simulink model "Vehicle_definitivo_validazione_2"  (R2025b)
settings: Solver=ode4  StartTime=0.0  StopTime=30  FixedStep=0.001  RelTol=1e-3
undefined symbols (not defined in the file): car, new_lotus_bump, new_lotus_roll, new_lotus_steer, posRef, rad, s, Tau_1, Tau_2, Tau_3, Tau_4, yawRef
libraries: aerolibconvert2 x28, simulink_extras x16, simulink x12, slpidlib x2, mpclib x1
(part 1 of 13)
settings Model: PacingRate=10  Creator=loren  LastModifiedBy=miche
settings SolverCC: ZeroCrossControl=DisableAll

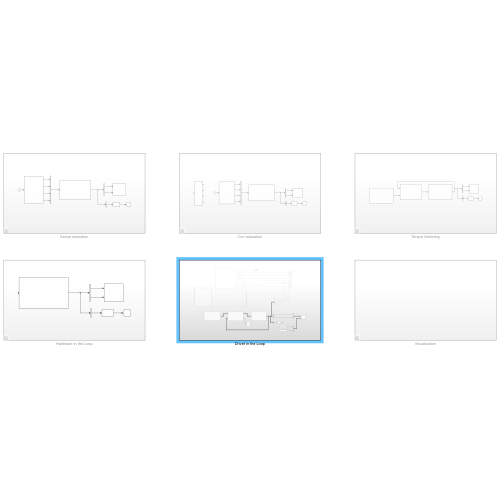
[thumbnail: Simulink's stored preview of the top-level diagram]
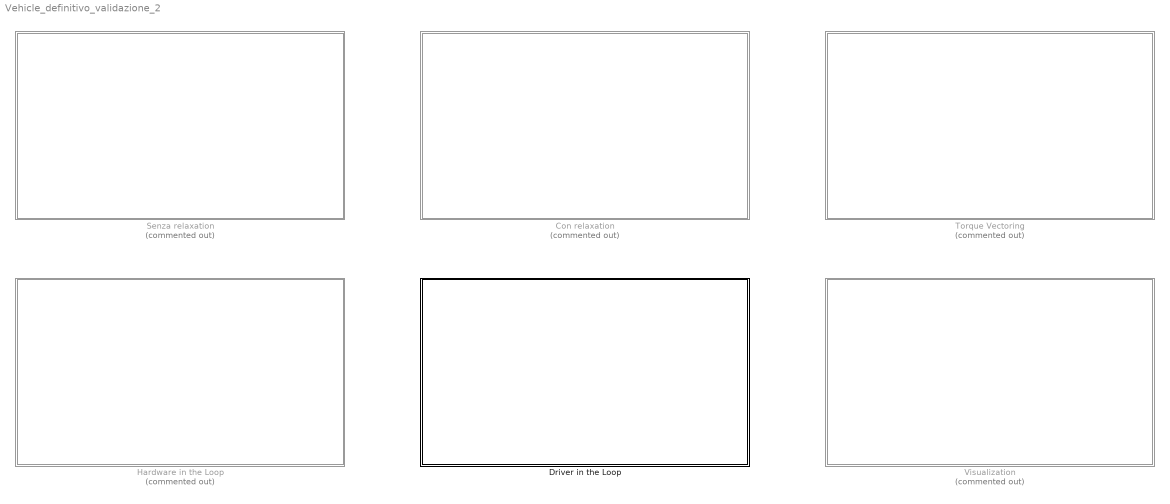
== system Vehicle_definitivo_validazione_2 ==
  Con relaxation : Subsystem  Commented=on
  Driver in the Loop : Subsystem
  Hardware in the Loop : Subsystem  Commented=on
  Senza relaxation : Subsystem  Commented=on
  Torque Vectoring : Subsystem  Commented=on
  Visualization : Subsystem  Commented=on

== system Vehicle_definitivo_validazione_2/Con relaxation ==
  Bus Creator : BusCreator  Inputs=4
  Bus Selector : BusSelector  OutputSignals=Veh_States.inertia_frame.X,Veh_States.inertia_frame.Y
  Bus Selector1 : BusSelector  OutputSignals=Veh_States.velocities.u
  Clock : Clock
  Compare To Constant3 : simulink/Logic and Bit Operations/Compare To Constant  relop=<=  const=2  OutDataTypeStr=boolean  ZeroCross=off
  MATLAB Function1 : MATLAB Function  TreatAsAtomicUnit=on
  MATLAB Function2 : MATLAB Function  TreatAsAtomicUnit=on
  Stop Simulation : Stop
  Vehicle : Subsystem
  XY Graph1 : Record  NumPorts=2.0  FileSettingsInternal="{\"entries\":[{\"content\":{\"excelSettings\":{\"content\":{},\"type\":\"Streamout.ExcelSettings\"},\"parquetSettings\":{\"content\":{},\"type\":\"Streamout.ParquetSettings\"}},\"type\":\"Streamout.FileSettingStorage\",\"uuid\":\"\"}],\"packageUris\":[\"http:\\/\\/schema.mathworks.com\\/mf0\\/streamout_blocks\\/R2020a\"],\"version\":\"1.0\"}"  FrameSettings=[0, 0]  Layout=[1 1]  SignalsInternal="{\"entries\":[{\"content\":{\"signals\":[{\"content\":{\"blockPath\":[],\"dimensions\":[1],\"domain\":\"\",\"lineColor\":\"#ff6929\",\"lineWidth\":2,\"port\":1,\"signalID\":1,\"signalName\":\"<X>\"},\"type\":\"RecordBlkView.Signal\",\"uuid\":\"\"},{\"content\":{\"blockPath\":[],\"dimensions\":[1],\"domain\":\"\",\"lineColor\":\"#b746ff\",\"lineWidth\":2,\"port\":2,\"signalID\":2,\"signalName\":\"<Y>\"},\"type\":\"RecordBlkView.Signal\",\"uuid\":\"\"}]},\"type\":\"RecordBlkView.InputSignals\",\"uuid\":\"\"}],\"packageUris\":[\"http:\\/\\/schema.mathworks.com\\/mf0\\/streamout_blocks\\/R2020a\"],\"version\":\"1.0\"}"  VisualizationBindings="{\"xyplotplugin\":{\"info\":[{\"series\":[],\"subplotID\":1}]}}"  CompatibilityTag=XY
  wires:
  Bus Creator/1 -> Vehicle/1(Driver)
  MATLAB Function2/4(bps) -> Bus Creator/4
  Clock/1 -> MATLAB Function2/1(t)
  MATLAB Function2/2(tps_ICE) -> Bus Creator/2
  Bus Selector1/1 -> Compare To Constant3/1  "<u>"
  MATLAB Function2/1(steer) -> Bus Creator/1
  Compare To Constant3/1 -> Stop Simulation/1
  Vehicle/1(Vehicle) -> Bus Selector1/1, Bus Selector/1  "Vehicle"
  MATLAB Function2/3(tps_EM) -> Bus Creator/3
  Bus Selector/1 -> XY Graph1/1  "<X>"
  Bus Selector/2 -> XY Graph1/2  "<Y>"

== system Vehicle_definitivo_validazione_2/Driver in the Loop ==
  Bus Creator : BusCreator  Inputs=2
  Bus Creator1 : BusCreator  Inputs=2
  Bus Creator2 : BusCreator  Commented=on  Inputs=4
  Bus Selector : BusSelector  OutputSignals=Veh_States.inertia_frame.X,Veh_States.inertia_frame.Y
  Bus Selector1 : BusSelector  OutputSignals=Veh_States.velocities.u
  Bus Selector2 : BusSelector  Commented=on  OutputSignals=Veh_States.velocities.u,Veh_States.accelerations.ax_prev,Veh_States.accelerations.ay_prev,Veh_States.velocities.v_tot
  Compare To Constant3 : simulink/Logic and Bit Operations/Compare To Constant  relop=<=  const=2  OutDataTypeStr=boolean  ZeroCross=off
  Constant : Constant  Commented=on  Value=0
  Constant1 : Constant  Commented=on  Value=0
  Driver : Subsystem
  From Workspace : FromWorkspace  VariableName=[t,posRef(:,1)]
  From Workspace1 : FromWorkspace  VariableName=[t,posRef(:,2)]
  From Spreadsheet : FromSpreadsheet  Commented=on  FileName=C:\Users\miche\Downloads\steer_fissato.xlsx  SheetName=Foglio1  Range=A3:H3989
  Gain : Gain  Commented=on  Gain=1/100
  Gain1 : Gain  Commented=on  Gain=-1
  Gain3 : Gain  Commented=on  Gain=1/3.6
  Gain4 : Gain  Commented=on  Gain=1/-9.81
  Gain7 : Gain  Commented=on  Gain=1/-9.81
  Lap Times : Display
  MATLAB Function versione 3 con memoria persistent1 : MATLAB Function  Commented=on  TreatAsAtomicUnit=on
  Scope : Scope
      settings: ActiveDisplayYMinimum=-1  ActiveDisplayYMaximum=1
  Scope1 : Scope  Commented=on
      settings: ActiveDisplayYMinimum=-1  ActiveDisplayYMaximum=1  DataLoggingVariableName=ScopeData6
  Scope2 : Scope  Commented=on
      settings: ActiveDisplayYMinimum=-89.125000000000455  ActiveDisplayYMaximum=-85.874999999999957  DataLoggingVariableName=ScopeData7
  Scope4 : Scope  Commented=on  NumInputPorts=3
      settings: ActiveDisplayYMinimum=2.9977159466940941  ActiveDisplayYMaximum=13.111056252836459  DataLoggingVariableName=ScopeData9
  Scope5 : Scope  Commented=on  NumInputPorts=2
      settings: ActiveDisplayYMinimum=-1.999530891220914  ActiveDisplayYMaximum=0.22217009902454593  DataLoggingVariableName=ScopeData10
  Scope6 : Scope  Commented=on  NumInputPorts=2
      settings: ActiveDisplayYMinimum=-1.1010446035915249  ActiveDisplayYMaximum=0.7997968068549437  DataLoggingVariableName=ScopeData11
  Stop Simulation : Stop
  Subsystem : Subsystem
  Terminator : Terminator
  Vehicle : Subsystem
  XY Graph : Record  NumPorts=2.0  FileSettingsInternal="{\"entries\":[{\"content\":{\"excelSettings\":{\"content\":{},\"type\":\"Streamout.ExcelSettings\"},\"parquetSettings\":{\"content\":{},\"type\":\"Streamout.ParquetSettings\"}},\"type\":\"Streamout.FileSettingStorage\",\"uuid\":\"\"}],\"packageUris\":[\"http:\\/\\/schema.mathworks.com\\/mf0\\/streamout_blocks\\/R2020a\"],\"version\":\"1.0\"}"  FrameSettings=[0, 0]  Layout=[1 1]  SignalsInternal="{\"entries\":[{\"content\":{\"signals\":[{\"content\":{\"blockPath\":[],\"dimensions\":[1],\"domain\":\"\",\"hasChildren\":true,\"lineColor\":\"#fe330a\",\"lineWidth\":2,\"port\":1,\"sid\":[\"\"],\"signalID\":1,\"signalName\":\"Bus\\nCreator\"},\"type\":\"RecordBlkView.Signal\",\"uuid\":\"\"},{\"content\":{\"blockPath\":[],\"dimensions\":[1],\"domain\":\"\",\"leafPath\":\"Bus\\nCreator.X\",\"lineColor\":\"#139fff\",\"lineWidth\":2,\"parentID\":1,\"plots\":[ 1 ],\"port\":1,\"sid\":[\"\"],\"signalID\":2,\"signalName\":\"Bus\\nCreator.X\"},\"type\":\"RecordBlkView.Signal\",\"uuid\":\"\"},{\"content\":{\"blockPath\":[],\"dimensions\":[1],\"domain\":\"\",\"leafPath\":\"Bus\\nCreator.Y\",\"lineColor\":\"#ff6929\",\"lineWidth\":2,\"parentID\":1,\"plots\":[ 1 ],\"port\":1,\"sid\":[\"\"],\"signalID\":3,\"signalName\":\"Bus\\nCreator.Y\"},\"type\":\"RecordBlkView.Signal\",\"uuid\":\"\"},{\"content\":{\"blockPath\":[],\"dimensions\":[1],\"domain\":\"\",\"hasChildren\":true,\"lineColor\":\"#d95319\",\"lineWidth\":2,\"port\":2,\"sid\":[\"\"],\"signalID\":4,\"signalName\":\"Bus\\nCreator1\"},\"type\":\"RecordBlkView.Signal\",\"uuid\":\"\"},{\"content\":{\"blockPath\":[],\"dimensions\":[1],\"domain\":\"\",\"leafPath\":\"Bus\\nCreator1.x_ref\",\"lineColor\":\"#fe330a\",\"lineWidth\":2,\"parentID\":4,\"plots\":[ 1 ],\"port\":2,\"sid\":[\"\"],\"signalID\":5,\"signalName\":\"Bus\\nCreator1.x_ref\"},\"type\":\"RecordBlkView.Signal\",\"uuid\":\"\"},{\"content\":{\"blockPath\":[],\"dimensions\":[1],\"domain\":\"\",\"leafPath\":\"Bus\\nCreator1.y_ref\",\"lineColor\":\"#22b573\",\"lineWidth\":2,\"parentID\":4,\"plots\":[ 1 ],\"port\":2,\"sid\":[\"\"],\"signalID\":6,\"signalName\":\"Bus\\nCreator1.y_ref\"},\"type\":\"RecordBlkView.Signal\",\"uuid\":\"\"}]},\"type\":\"RecordBlkView.InputSignals\",\"uuid\":\"\"}],\"packageUris\":[\"http:\\/\\/schema.mathworks.com\\/mf0\\/streamout_blocks\\/R2020a\"],\"version\":\"1.0\"}"  VisualizationBindings="{\"xyplotplugin\":{\"info\":[{\"series\":[{\"bindingParametersList\":[{\"parameter\":\"X-Axis\",\"signalID\":2,\"signalName\":\"Bus\\nCreator.X\"},{\"parameter\":\"Y-Axis\",\"signalID\":3,\"signalName\":\"Bus\\nCreator.Y\"}],\"seriesID\":0},{\"bindingParametersList\":[{\"parameter\":\"X-Axis\",\"signalID\":5,\"signalName\":\"Bus\\nCreator1.x_ref\"},{\"parameter\":\"Y-Axis\",\"signalID\":6,\"signalName\":\"Bus\\nCreator1.y_ref\"}],\"seriesID\":1}],\"subplotID\":1}]}}"  CompatibilityTag=XY
  wires:
  Bus Selector/2 -> Bus Creator/2  "<Y>"
  Bus Selector1/1 -> Compare To Constant3/1  "<u>"
  Compare To Constant3/1 -> Stop Simulation/1
  Bus Selector/1 -> Bus Creator/1  "<X>"
  Vehicle/1(Vehicle) -> Driver/2(Feedback), Bus Selector1/1, Bus Selector2/1, Bus Selector/1  "Vehicle"
  Subsystem/1(Reference) -> Driver/1(Reference)
  Driver/2(LapTimes) -> Lap Times/1
  From Workspace1/1 -> Bus Creator1/2  "y_ref"
  From Workspace/1 -> Bus Creator1/1  "x_ref"
  Bus Creator/1 -> XY Graph/1
  From Spreadsheet/4 -> Gain1/1
  Gain/1 -> Bus Creator2/2, Scope1/1  "tps_ICE"
  Constant1/1 -> Bus Creator2/3  "tps_EM"
  Constant/1 -> Bus Creator2/4  "bps"
  From Spreadsheet/1 -> Terminator/1  "gear"
  From Spreadsheet/2 -> Scope/1  "engine speed"
  From Spreadsheet/3 -> Gain/1
  From Spreadsheet/7 -> Scope6/1  "G long"
  From Spreadsheet/6 -> Scope5/1  "G lat"
  From Spreadsheet/5 -> Gain3/1  "gps speed"
  Gain1/1 -> Bus Creator2/1, Scope2/1  "steer"
  Bus Creator1/1 -> XY Graph/2
  Bus Selector2/2 -> Gain7/1  "<ax_prev>"
  Bus Selector2/3 -> Gain4/1  "<ay_prev>"
  Bus Selector2/1 -> Scope4/2  "<u>"
  Bus Selector2/4 -> Scope4/3  "<v_tot>"
  Gain3/1 -> Scope4/1  "gps speed"
  Gain7/1 -> Scope6/2  "G lat"
  Gain4/1 -> Scope5/2  "G lat"
  Driver/1(Driver) -> Vehicle/1(Driver)  "Driver"

== system Vehicle_definitivo_validazione_2/Hardware in the Loop ==
  Bus Selector : BusSelector  OutputSignals=Veh_States.inertia_frame.X,Veh_States.inertia_frame.Y
  Bus Selector1 : BusSelector  OutputSignals=Veh_States.velocities.u
  Compare To Constant3 : simulink/Logic and Bit Operations/Compare To Constant  relop=<=  const=2  OutDataTypeStr=boolean  ZeroCross=off
  Stop Simulation : Stop
  Vehicle : Subsystem
  XY Graph1 : Record  NumPorts=2.0  FileSettingsInternal="{\"entries\":[{\"content\":{\"excelSettings\":{\"content\":{},\"type\":\"Streamout.ExcelSettings\"},\"parquetSettings\":{\"content\":{},\"type\":\"Streamout.ParquetSettings\"}},\"type\":\"Streamout.FileSettingStorage\",\"uuid\":\"\"}],\"packageUris\":[\"http:\\/\\/schema.mathworks.com\\/mf0\\/streamout_blocks\\/R2020a\"],\"version\":\"1.0\"}"  FrameSettings=[0, 0]  Layout=[1 1]  SignalsInternal="{\"entries\":[{\"content\":{\"signals\":[{\"content\":{\"blockPath\":[],\"dimensions\":[1],\"domain\":\"\",\"lineColor\":\"#22b573\",\"lineWidth\":2,\"port\":1,\"signalID\":1,\"signalName\":\"<X>\"},\"type\":\"RecordBlkView.Signal\",\"uuid\":\"\"},{\"content\":{\"blockPath\":[],\"dimensions\":[1],\"domain\":\"\",\"lineColor\":\"#0072bd\",\"lineWidth\":2,\"port\":2,\"signalID\":2,\"signalName\":\"<Y>\"},\"type\":\"RecordBlkView.Signal\",\"uuid\":\"\"}]},\"type\":\"RecordBlkView.InputSignals\",\"uuid\":\"\"}],\"packageUris\":[\"http:\\/\\/schema.mathworks.com\\/mf0\\/streamout_blocks\\/R2020a\"],\"version\":\"1.0\"}"  VisualizationBindings="{\"xyplotplugin\":{\"info\":[{\"series\":[],\"subplotID\":1}]}}"  CompatibilityTag=XY
  wires:
  Bus Selector/2 -> XY Graph1/2  "<Y>"
  Bus Selector1/1 -> Compare To Constant3/1  "<u>"
  Compare To Constant3/1 -> Stop Simulation/1
  Bus Selector/1 -> XY Graph1/1  "<X>"
  Vehicle/1(Vehicle) -> Bus Selector1/1, Bus Selector/1  "Vehicle"

== system Vehicle_definitivo_validazione_2/Senza relaxation ==
  Bus Creator : BusCreator  Inputs=4
  Bus Selector2 : BusSelector  OutputSignals=Veh_States.inertia_frame.X,Veh_States.inertia_frame.Y
  Bus Selector3 : BusSelector  OutputSignals=Veh_States.velocities.u
  Clock : Clock
  Compare To Constant1 : simulink/Logic and Bit Operations/Compare To Constant  relop=<=  const=2  OutDataTypeStr=boolean  ZeroCross=off
  MATLAB Function2 : MATLAB Function  TreatAsAtomicUnit=on
  Stop Simulation1 : Stop
  Vehicle : Subsystem
  XY Graph2 : Record  NumPorts=2.0  FileSettingsInternal="{\"entries\":[{\"content\":{\"excelSettings\":{\"content\":{},\"type\":\"Streamout.ExcelSettings\"},\"parquetSettings\":{\"content\":{},\"type\":\"Streamout.ParquetSettings\"}},\"type\":\"Streamout.FileSettingStorage\",\"uuid\":\"\"}],\"packageUris\":[\"http:\\/\\/schema.mathworks.com\\/mf0\\/streamout_blocks\\/R2020a\"],\"version\":\"1.0\"}"  FrameSettings=[0, 0]  Layout=[1 1]  SignalsInternal="{\"entries\":[{\"content\":{},\"type\":\"RecordBlkView.InputSignals\",\"uuid\":\"\"}],\"packageUris\":[\"http:\\/\\/schema.mathworks.com\\/mf0\\/streamout_blocks\\/R2020a\"],\"version\":\"1.0\"}"  VisualizationBindings="{\"xyplotplugin\":{\"info\":[{\"series\":[],\"subplotID\":1}]}}"  CompatibilityTag=XY
  wires:
  Vehicle/1(Vehicle) -> Bus Selector3/1, Bus Selector2/1  "Vehicle"
  Compare To Constant1/1 -> Stop Simulation1/1
  Bus Selector3/1 -> Compare To Constant1/1  "<u>"
  MATLAB Function2/2(tps_ICE) -> Bus Creator/2
  MATLAB Function2/3(tps_EM) -> Bus Creator/3
  Clock/1 -> MATLAB Function2/1(t)
  MATLAB Function2/4(bps) -> Bus Creator/4
  MATLAB Function2/1(steer) -> Bus Creator/1
  Bus Creator/1 -> Vehicle/1(Driver)
  Bus Selector2/1 -> XY Graph2/1  "<X>"
  Bus Selector2/2 -> XY Graph2/2  "<Y>"

== system Vehicle_definitivo_validazione_2/Torque Vectoring ==
  Bus Selector4 : BusSelector  OutputSignals=Veh_States.inertia_frame.X,Veh_States.inertia_frame.Y
  Bus Selector5 : BusSelector  OutputSignals=Veh_States.velocities.u
  Compare To Constant2 : simulink/Logic and Bit Operations/Compare To Constant  relop=<=  const=2  OutDataTypeStr=boolean  ZeroCross=off
  Driver : Subsystem
  Stop Simulation2 : Stop
  Vehicle : Subsystem
  Vehicle Control Unit : Subsystem
  XY Graph3 : Record  NumPorts=2.0  FileSettingsInternal="{\"entries\":[{\"content\":{\"excelSettings\":{\"content\":{},\"type\":\"Streamout.ExcelSettings\"},\"parquetSettings\":{\"content\":{},\"type\":\"Streamout.ParquetSettings\"}},\"type\":\"Streamout.FileSettingStorage\",\"uuid\":\"\"}],\"packageUris\":[\"http:\\/\\/schema.mathworks.com\\/mf0\\/streamout_blocks\\/R2020a\"],\"version\":\"1.0\"}"  FrameSettings=[0, 0]  Layout=[1 1]  SignalsInternal="{\"entries\":[{\"content\":{},\"type\":\"RecordBlkView.InputSignals\",\"uuid\":\"\"}],\"packageUris\":[\"http:\\/\\/schema.mathworks.com\\/mf0\\/streamout_blocks\\/R2020a\"],\"version\":\"1.0\"}"  VisualizationBindings="{\"xyplotplugin\":{\"info\":[{\"series\":[],\"subplotID\":1}]}}"  CompatibilityTag=XY
  wires:
  Vehicle/1(Vehicle) -> Bus Selector5/1, Bus Selector4/1, Vehicle Control Unit/1(Vehicle)  "Vehicle"
  Vehicle Control Unit/1(Driver_out) -> Vehicle/1(Driver)
  Bus Selector5/1 -> Compare To Constant2/1  "<u>"
  Compare To Constant2/1 -> Stop Simulation2/1
  Driver/1(Driver) -> Vehicle Control Unit/2(Driver_in)
  Bus Selector4/2 -> XY Graph3/2  "<Y>"
  Bus Selector4/1 -> XY Graph3/1  "<X>"

== system Vehicle_definitivo_validazione_2/Visualization ==

== system Vehicle_definitivo_validazione_2/Con relaxation/Vehicle ==
  Driver : Inport
  Brakes : Subsystem
  Bus Selector : BusSelector  OutputSignals=steer,tps_ICE,tps_EM,bps
  Chassis : Subsystem
  Powertrain : Subsystem
  Solver : Subsystem
  Tyres : Subsystem
  Vehicle : Outport
  wires:
  Driver/1 -> Bus Selector/1
  Tyres/1(omega_wheels) -> Powertrain/2(omega_wheels)
  Brakes/1(Brake_torque) -> Tyres/3(T_brake)
  Bus Selector/1 -> Chassis/2(<steer>)  "<steer>"
  Chassis/1(forces & kinematics) -> Solver/1(forces & kinematics), Tyres/1(forces & kinematics)
  Chassis/2(J) -> Tyres/4(J)
  Bus Selector/2 -> Powertrain/1(tps_ICE)  "<tps_ICE>"
  Powertrain/1(gear) -> Chassis/3(gear)
  Powertrain/2(torque) -> Tyres/2(T_motor)
  Tyres/2(Tire_Forces) -> Solver/2(Tire_Forces)
  Solver/1(Vehicle) -> Vehicle/1, Powertrain/3(vehicle), Tyres/5(Vehicle), Chassis/1(Veh_States)
  Bus Selector/4 -> Brakes/1(BP_tot), Powertrain/5(bps)  "<bps>"
  Bus Selector/3 -> Powertrain/4(tps_EM)  "<tps_EM>"

== system Vehicle_definitivo_validazione_2/Driver in the Loop/Driver ==
  Reference : Inport
  Feedback : Inport  Port=2
  Average Time : Display
  Bus Creator : BusCreator  Inputs=5
  Bus Selector1 : BusSelector  OutputSignals=x_ref,y_ref,yaw ref,vtot_target
  Bus Selector2 : BusSelector  OutputSignals=Veh_States.inertia_frame.X,Veh_States.inertia_frame.Y,Veh_States.inertia_frame.yaw,Veh_States.velocities.u,Veh_States.velocities.v,Veh_States.velocities.r,Veh_States.velocities.v_tot,Torque_rear.T_RR,Torque_rear.T_RL
  Clock : Clock
  Compare To Constant3 : simulink/Logic and Bit Operations/Compare To Constant  relop=>=  const=30  OutDataTypeStr=boolean  ZeroCross=off
  Constant : Constant  Value=2
  Constant1 : Constant  Value=[0;0;0;0]
  Constant3 : Constant  Value=0
  Constant4 : Constant  Commented=on  Value=car  OutDataTypeStr=Bus: slBus1
  Constant9 : Constant  Value=car  OutDataTypeStr=Bus: slBus1
  Current Lap : Display
  Divide : Product  Inputs=*/
  Gain : Gain  Gain=-1
  Lap Time Counter : MATLAB Function  TreatAsAtomicUnit=on
  MATLAB Function versione 4 con memoria persistent : MATLAB Function  TreatAsAtomicUnit=on
  MATLAB Function1 : MATLAB Function  Commented=on  TreatAsAtomicUnit=on
  MPC Controller1 : mpclib/MPC Controller  SCDEnableBlockLinearizationSpecification=on  mpcobj=mpcobj_dyn  is_multiple=0  enable_value=0  return_u0=off  updateMPCinCallerWorkspace=on  md_inport=on  mv_inport=off  uref_inport=off  return_cost=off  return_mvseq=off  return_qpstatus=off  return_xseq=off  return_state=off  return_ovseq=off  state_inport=off  umin_inport=off  umax_inport=off  ymin_inport=off  ymax_inport=off  cc_inport=off  ywt_inport=off  uwt_inport=off  duwt_inport=off  rhoeps_inport=off  pm_inport=off  MaximumP=10  HorizonChoice=FixedHorizon  n_ts=0.005  n_p=100  n_mv=1  n_md=2  n_ud=0  n_mo=4  n_uo=0  BlockDataType=double  SampleTimeInherited=off  switch_inport=off
  Mux : Mux  Inputs=2
  Mux1 : Mux
  PID Controller : slpidlib/PID Controller  Controller=PI  Form=Parallel  TimeDomain=Continuous-time  UseExternalTs=off  SampleTime=-1  IntegratorMethod=Forward Euler  FilterMethod=Forward Euler  ControllerParametersSource=internal  P=5  I=5  UseKiTs=off  D=5  UseExternalDerivativeSource=off  N=70870.8659161454  UseFilter=on  TunerSelectOption=Transfer Function Based (PID Tuner App)  InitialConditionSource=internal  InitialConditionForIntegrator=0  InitialConditionForFilter=0  DifferentiatorICPrevScaledInput=0  ExternalReset=none  TrackingMode=off  Kt=1  LimitOutput=on  SatLimitsSource=internal  UpperSaturationLimit=1  LowerSaturationLimit=-1  LinearizeAsGain=on  AntiWindupMode=clamping  Kb=1  LimitIntegrator=off  UpperIntegratorSaturationLimit=inf  LowerIntegratorSaturationLimit=-inf  POutMin=[]  POutMax=[]  IOutMin=[]  IOutMax=[]  DOutMin=[]  DOutMax=[]  NOutMin=[]  NOutMax=[]  SumOutMin=[]  SumOutMax=[]  SaturationOutMin=[]  SaturationOutMax=[]  PParamMin=[]  PParamMax=[]  IParamMin=[]  IParamMax=[]  DParamMin=[]  DParamMax=[]  NParamMin=[]  NParamMax=[]  KbParamMin=[]  KbParamMax=[]  KtParamMin=[]  KtParamMax=[]  KbOutMin=[]  KbOutMax=[]  KtOutMin=[]  KtOutMax=[]  IntegratorOutMin=[]  IntegratorOutMax=[]  FilterOutMin=[]  FilterOutMax=[]  SumI1OutMin=[]  SumI1OutMax=[]  SumI2OutMin=[]  SumI2OutMax=[]  SumI3OutMin=[]  SumI3OutMax=[]  SumI4OutMin=[]  SumI4OutMax=[]  SumDOutMin=[]  SumDOutMax=[]  DifferentiatorOutMin=[]  DifferentiatorOutMax=[]  FilterDiffOutCoefMin=[]  FilterDiffOutCoefMax=[]  ReciprocalOutMin=[]  ReciprocalOutMax=[]  SumDenOutMin=[]  SumDenOutMax=[]  SumNumOutMin=[]  SumNumOutMax=[]  DivideOutMin=[]  DivideOutMax=[]  UdiffTsProdOutMin=[]  UdiffTsProdOutMax=[]  NTsProdOutMin=[]  NTsProdOutMax=[]  UintegralTsProdOutMin=[]  UintegralTsProdOutMax=[]  UngainTsProdOutMin=[]  UngainTsProdOutMax=[]  ClampingZeroOutDataTypeStr=Inherit: Inherit via back propagation  ClampingZeroOutMin=[]  ClampingZeroOutMax=[]  FilterDenConstantOutDataTypeStr=Inherit: Inherit via back propagation  FilterDenConstantOutMin=[]  FilterDenConstantOutMax=[]  PCopyOutDataTypeStr=Inherit: Inherit via back propagation  PCopyOutMin=[]  PCopyOutMax=[]  NCopyOutDataTypeStr=Inherit: Inherit via back propagation  NCopyOutMin=[]  NCopyOutMax=[]  IntegratorContinuousStateAttributes=''  IntegratorStateMustResolveToSignalObject=off  IntegratorRTWStateStorageClass=Auto  FilterContinuousStateAttributes=''  FilterStateMustResolveToSignalObject=off  FilterRTWStateStorageClass=Auto  ParallelPVariant=InternalParameters  IdealPVariant=Disabled  IVariant=InternalParameters  DVariant=Disabled  IntegratorVariant=Continuous  SatVariant=Enabled  AWVariant=ContClampingParallel  PCopyVariant=Disabled  TRVariant=Disabled  FdbkBlocksVariant=Forward  IdealPFdbkVariant=Disabled  SatFdbkVariant=Disabled  DerivativeFilterVariant=Disabled  NVariant=Disabled  NCopyVariant=Disabled_SignalSpec  FilterICVariant=Disabled  IntegratorICVariant=InternalICs  ExternalResetVariant=Disabled  TRSumVariant=Passthrough  SumFdbkVariant=Disabled  SumVariant=Sum_PI  TsampFilterVariant=InternalTs  TsampNgainVariant=Passthrough  TsampIntegralVariant=Disabled_SignalSpec  ExternalSaturationOutDataTypeStr=Inherit: Same as second input  DerivativeSourceVariant=Disabled  PreIntVariant=InternalPreInt
  Saturation : Saturate  UpperLimit=1  LowerLimit=0
  Saturation1 : Saturate  UpperLimit=1  LowerLimit=0
  Saturation2 : Saturate  UpperLimit=6  LowerLimit=1  ZeroCross=off
  Scope : Scope
      settings: ActiveDisplayYMinimum=-2.2641954274492662  ActiveDisplayYMaximum=3.3543848288211962
  Scope1 : Scope
      settings: ActiveDisplayYMinimum=-0.18062887327134342  ActiveDisplayYMaximum=0.067368300453348545  DataLoggingVariableName=ScopeData2
  Scope3 : Scope
      settings: ActiveDisplayYMinimum=0.049977073798069746  ActiveDisplayYMaximum=0.1226811189845797  DataLoggingVariableName=ScopeData4
  Stop Simulation : Stop
  Subtract : Sum  Inputs=+-
  Sum of Elements : Sum  Inputs=+
  Driver : Outport
  LapTimes : Outport  Port=2
  wires:
  Reference/1 -> Bus Selector1/1
  Bus Selector1/4 -> Subtract/1  "<vtot_target>"
  Subtract/1 -> PID Controller/1  "target"
  Gain/1 -> Saturation1/1
  Saturation1/1 -> Bus Creator/5  "bps"
  Saturation/1 -> Bus Creator/3  "tps_ICE"
  Bus Creator/1 -> Driver/1
  Constant/1 -> Bus Creator/2  "gear"
  Bus Selector1/1 -> MATLAB Function versione 4 con memoria persistent/8(X_ref)  "<x_ref>"
  Bus Selector1/3 -> MATLAB Function versione 4 con memoria persistent/10(psi_ref)  "<yaw ref>"
  Bus Selector1/2 -> MATLAB Function versione 4 con memoria persistent/9(Y_ref)  "<y_ref>"
  Feedback/1 -> Bus Selector2/1
  Bus Selector2/1 -> [x_car], MATLAB Function versione 4 con memoria persistent/2(X_car)  "<X>"
  Bus Selector2/2 -> [y_car], MATLAB Function versione 4 con memoria persistent/3(Y_car)  "<Y>"
  Bus Selector2/3 -> MATLAB Function versione 4 con memoria persistent/4(psi_car)  "<yaw>"
  Bus Selector2/4 -> MATLAB Function versione 4 con memoria persistent/5(u_car)  "<u>"
  Bus Selector2/5 -> MATLAB Function versione 4 con memoria persistent/6(v_y_car)  "<v>"
  Bus Selector2/6 -> MATLAB Function versione 4 con memoria persistent/7(r_car)  "<r>"
  MATLAB Function versione 4 con memoria persistent/1(e_y) -> Scope1/1, Mux1/1  "lateral error"
  Mux1/1 -> MPC Controller1/1
  MATLAB Function versione 4 con memoria persistent/2(e_y_dot) -> Mux1/2  "lateral error derivative"
  MATLAB Function versione 4 con memoria persistent/3(e_psi) -> Scope3/1, Mux1/3  "yaw angle error"
  MPC Controller1/1 -> Scope/1, Bus Creator/1  "steer"
  Constant1/1 -> MPC Controller1/2
  Bus Selector2/7 -> Subtract/2  "<v_tot>"
  Lap Time Counter/2(CurrLapNum) -> Saturation2/1
  Clock/1 -> Lap Time Counter/3(t)  "t"
  Saturation2/1 -> Current Lap/1, Divide/2
  [x_car] -> Compare To Constant3/1, Lap Time Counter/1(X)  "x"
  Divide/1 -> Average Time/1
  [y_car] -> Lap Time Counter/2(Y)  "y"
  Sum of Elements/1 -> Divide/1
  Lap Time Counter/1(LapTimes) -> Sum of Elements/1, LapTimes/1
  Compare To Constant3/1 -> Stop Simulation/1
  MATLAB Function versione 4 con memoria persistent/4(e_psi_dot) -> Mux1/4  "yaw derivative"
  MATLAB Function versione 4 con memoria persistent/5(psi_dot_res_out) -> Mux/1  "psi_dot_res_out"
  PID Controller/1 -> Gain/1, Saturation/1
  Constant3/1 -> Bus Creator/4  "tps_EM"
  Mux/1 -> MPC Controller1/3
  Bus Selector2/8 -> MATLAB Function versione 4 con memoria persistent/11(T_RR)  "<T_RR>"
  Bus Selector2/9 -> MATLAB Function versione 4 con memoria persistent/12(T_RL)  "<T_RL>"
  MATLAB Function versione 4 con memoria persistent/6(Mz_lsd) -> Mux/2  "Mz_lsd"
  Constant9/1 -> MATLAB Function versione 4 con memoria persistent/1(car)
  Constant4/1 -> MATLAB Function1/2(gear)
  ? -> MATLAB Function1/1(v_target)  "<vtot_target>"

== system Vehicle_definitivo_validazione_2/Driver in the Loop/Subsystem ==
  Bus Creator : BusCreator  Inputs=4
  Constant : Constant  Value=posRef(:,1)
  Constant1 : Constant  Value=posRef(:,2)
  Constant2 : Constant  Value=deg2rad(yawRef)
  Constant3 : Constant  Value=34/3.6
  Reference : Outport
  wires:
  Constant3/1 -> Bus Creator/4  "vtot_target"
  Bus Creator/1 -> Reference/1
  Constant/1 -> Bus Creator/1  "x_ref"
  Constant1/1 -> Bus Creator/2  "y_ref"
  Constant2/1 -> Bus Creator/3  "yaw ref"

== system Vehicle_definitivo_validazione_2/Driver in the Loop/Vehicle ==
  Driver : Inport
  Brakes : Subsystem
  Bus Selector : BusSelector  OutputSignals=steer,tps_ICE,tps_EM,bps
  Chassis : Subsystem
  Powertrain : Subsystem
  Radians to Degrees : simulink_extras/Transformations/Radians to Degrees
  Solver : Subsystem
  Tyres1 con relaxation : Subsystem  Commented=on
  Tyres1 senza relaxation : Subsystem
  Vehicle : Outport
  wires:
  Driver/1 -> Bus Selector/1
  Tyres1 senza relaxation/1(omega_wheels) -> Powertrain/2(omega_wheels)
  Brakes/1(Brake_torque) -> Tyres1 senza relaxation/3(T_brake)
  Bus Selector/1 -> Radians to Degrees/1  "<steer>"
  Chassis/1(forces & kinematics) -> Tyres1 senza relaxation/1(forces & kinematics), Solver/1(forces & kinematics)
  Chassis/2(J) -> Tyres1 senza relaxation/4(J)
  Bus Selector/2 -> Powertrain/1(tps_ICE)  "<tps_ICE>"
  Powertrain/1(gear) -> Chassis/3(gear)
  Powertrain/2(torque) -> [T_rear], Tyres1 senza relaxation/2(T_motor)
  Tyres1 senza relaxation/2(Tire_Forces) -> Solver/2(Tire_Forces)
  Solver/1(Vehicle) -> Vehicle/1, Chassis/1(Veh_States), Tyres1 senza relaxation/5(Veh_States), Powertrain/3(vehicle)
  Bus Selector/4 -> Brakes/1(BP_tot), Powertrain/5(bps)  "<bps>"
  Bus Selector/3 -> Powertrain/4(tps_EM)  "<tps_EM>"
  [T_rear] -> Solver/3(T_rear)
  Radians to Degrees/1 -> Chassis/2(<steer>)

== system Vehicle_definitivo_validazione_2/Hardware in the Loop/Vehicle ==
  Driver : Inport
  Brakes : Subsystem
  Bus Selector : BusSelector  OutputSignals=steer,tps_ICE,tps_EM,bps
  Chassis : Subsystem
  Powertrain : Subsystem
  Solver : Subsystem
  Tyres : Subsystem
  Vehicle : Outport
  wires:
  Driver/1 -> Bus Selector/1
  Tyres/1(omega_wheels) -> Powertrain/2(omega_wheels)
  Brakes/1(Brake_torque) -> Tyres/3(T_brake)
  Bus Selector/1 -> Chassis/2(<steer>)  "<steer>"
  Chassis/1(forces & kinematics) -> Solver/1(forces & kinematics), Tyres/1(forces & kinematics)
  Chassis/2(J) -> Tyres/4(J)
  Bus Selector/2 -> Powertrain/1(tps_ICE)  "<tps_ICE>"
  Powertrain/1(gear) -> Chassis/3(gear)
  Powertrain/2(torque) -> Tyres/2(T_motor)
  Tyres/2(Tire_Forces) -> Solver/2(Tire_Forces)
  Solver/1(Vehicle) -> Vehicle/1, Powertrain/3(vehicle), Tyres/5(Vehicle), Chassis/1(Veh_States)
  Bus Selector/4 -> Brakes/1(BP_tot), Powertrain/5(bps)  "<bps>"
  Bus Selector/3 -> Powertrain/4(tps_EM)  "<tps_EM>"

== system Vehicle_definitivo_validazione_2/Senza relaxation/Vehicle ==
  Driver : Inport
  Brakes : Subsystem
  Bus Selector : BusSelector  OutputSignals=steer,tps_ICE,tps_EM,bps
  Chassis : Subsystem
  Powertrain : Subsystem
  Solver : Subsystem
  Tyres : Subsystem
  Vehicle : Outport
  wires:
  Driver/1 -> Bus Selector/1
  Tyres/1(omega_wheels) -> Powertrain/2(omega_wheels)
  Brakes/1(Brake_torque) -> Tyres/3(T_brake)
  Bus Selector/1 -> Chassis/2(<steer>)  "<steer>"
  Chassis/1(forces & kinematics) -> Tyres/1(forces & kinematics), Solver/1(forces & kinematics)
  Chassis/2(J) -> Tyres/4(J)
  Bus Selector/2 -> Powertrain/1(tps_ICE)  "<tps_ICE>"
  Powertrain/1(gear) -> Chassis/3(gear)
  Powertrain/2(torque) -> Tyres/2(T_motor)
  Tyres/2(Tire_Forces) -> Solver/2(Tire_Forces)
  Solver/1(Vehicle) -> Chassis/1(Veh_States), Powertrain/3(vehicle), Tyres/5(Veh_States), Vehicle/1
  Bus Selector/4 -> Powertrain/5(bps), Brakes/1(BP_tot)  "<bps>"
  Bus Selector/3 -> Powertrain/4(tps_EM)  "<tps_EM>"

== system Vehicle_definitivo_validazione_2/Torque Vectoring/Driver ==
  Bus Creator2 : BusCreator  Inputs=3
  Clock : Clock
  Constant : Constant
  Constant1 : Constant  Value=0
  Constant2 : Constant  Value=0
  MATLAB Function3 : MATLAB Function  TreatAsAtomicUnit=on
  Driver : Outport
  wires:
  Bus Creator2/1 -> Driver/1
  Clock/1 -> MATLAB Function3/1(t)
  Constant/1 -> ?  "tps_ICE"
  Constant2/1 -> ?  "bps"
  Constant1/1 -> ?  "steer"
  MATLAB Function3/1(steer) -> Bus Creator2/1
  MATLAB Function3/2(tps_ICE) -> Bus Creator2/2
  MATLAB Function3/3(bps) -> Bus Creator2/3

== system Vehicle_definitivo_validazione_2/Torque Vectoring/Vehicle ==
  Driver : Inport
  Brakes : Subsystem
  Bus Selector : BusSelector  OutputSignals=Driver_in.steer,Driver_in.tps_ICE,T_target,Driver_in.bps
  Chassis : Subsystem
  Powertrain : Subsystem
  Powertrain con differenziale1 : Subsystem  Commented=on
  Solver : Subsystem
  Tyres : Subsystem
  Vehicle : Outport
  wires:
  Driver/1 -> Bus Selector/1
  Tyres/1(omega_wheels) -> Powertrain/2(omega_wheels)
  Brakes/1(Brake_torque) -> Tyres/3(T_brake)
  Chassis/1(forces & kinematics) -> Solver/1(forces & kinematics), Tyres/1(forces & kinematics)
  Chassis/2(J) -> Tyres/4(J)
  Powertrain/1(gear) -> Chassis/3(gear)
  Powertrain/2(torque) -> Tyres/2(T_motor)
  Tyres/2(Tire_Forces) -> Solver/2(Tire_Forces)
  Solver/1(Vehicle) -> Chassis/1(Veh_States), Powertrain/3(vehicle), Tyres/5(Vehicle), Vehicle/1
  Bus Selector/1 -> Chassis/2(<steer>)  "<steer>"
  Bus Selector/2 -> Powertrain/1(tps_ICE)  "<tps_ICE>"
  Bus Selector/3 -> Powertrain/4(T_target)  "<T_target>"
  Bus Selector/4 -> Powertrain/5(bps), Brakes/1(BP_tot)  "<bps>"

== system Vehicle_definitivo_validazione_2/Torque Vectoring/Vehicle Control Unit ==
  Vehicle : Inport
  Driver_in : Inport  Port=2
  Bus Creator : BusCreator  Inputs=2
  High Level Controller : Subsystem
  Low Level Controller : Subsystem
  Torque Allocator : Subsystem
  Driver_out : Outport
  wires:
  Vehicle/1 -> High Level Controller/1(Vehicle), Low Level Controller/1(Vehicle)
  Driver_in/1 -> Torque Allocator/2(Driver_in), Bus Creator/1, High Level Controller/2(Driver_in)  "Driver_in"
  High Level Controller/1(Mz_delta) -> Torque Allocator/1(Mz_delta)
  Torque Allocator/1(T_front) -> Low Level Controller/2(T_front)
  Low Level Controller/1(T_target) -> Bus Creator/2  "T_target"
  Bus Creator/1 -> Driver_out/1  "Driver_out"

== system Vehicle_definitivo_validazione_2/Con relaxation/Vehicle/Brakes ==
  BP_tot : Inport
  Constant : Constant  Value=car.bp_max
  Front Caliper : Subsystem
  Gain : Gain  Gain=car.brakebias
  Gain1 : Gain  Gain=1-car.brakebias
  Mux : Mux
  Product2 : Product
  Proportional Valve : Subsystem
  Rear Caliper : Subsystem
  Brake_torque : Outport
  wires:
  Gain/1 -> Front Caliper/1(P_Front)
  Proportional Valve/1(p_rear_mod) -> Rear Caliper/1(P_rear)
  Gain1/1 -> Proportional Valve/1(P_rear)
  Product2/1 -> Gain1/1, Gain/1
  Rear Caliper/1(T_brake_RR) -> Mux/3  "T_brake_RR"
  Rear Caliper/2(T_brake_RL) -> Mux/4  "T_brake_RL"
  Mux/1 -> Brake_torque/1  "Brake_Torque"
  BP_tot/1 -> Product2/1
  Constant/1 -> Product2/2
  Front Caliper/2(T_brake_FL) -> Mux/2  "T_brake_FL"
  Front Caliper/1(T_brake_FR) -> Mux/1  "T_brake_FR"

== system Vehicle_definitivo_validazione_2/Con relaxation/Vehicle/Chassis ==
  Veh_States : Inport
  <steer> : Inport  Port=2
  gear : Inport  Port=3
  Aeromaps : Subsystem
  Bus Creator : BusCreator  Inputs=3
  Bus Creator1 : BusCreator  Inputs=2
  Bus Creator2 : BusCreator  Inputs=2
  Bus Selector : BusSelector  OutputSignals=Veh_States.accelerations.ax_prev,Veh_States.accelerations.ay_prev,Veh_States.velocities.u
  Constant : Constant  Value=0
  Constant12 : Constant  Value=car  OutDataTypeStr=Bus: slBus1
  Constant5 : Constant  Value=car.J_f
  Damper : Subsystem
  Integrator4 : Integrator  InitialCondition=zeros(14,1)
  MATLAB Function4 : MATLAB Function  TreatAsAtomicUnit=on
  MATLAB Function5 : MATLAB Function  TreatAsAtomicUnit=on
  Memory2 : Memory  InheritSampleTime=on
  Memory3 : Memory  InitialCondition=[car.Cz, car.Cx, car.x_cp]  InheritSampleTime=on
  Memory5 : Memory  InitialCondition=[car.IR_spring_front, car.IR_spring_front, car.IR_spring_rear, car.IR_spring_rear, car.tf, car.tr, car.lf, car.lr, car.h_cog, 0.03, 0.04]  InheritSampleTime=on
  Mux : Mux
  Mux2 : Mux
  Terminator : Terminator
  kinematics : Subsystem
  forces & kinematics : Outport
  J : Outport  Port=2
  wires:
  MATLAB Function5/1(dx) -> Integrator4/1
  gear/1 -> MATLAB Function4/1(gear)
  Constant12/1 -> MATLAB Function4/2(car), MATLAB Function5/9(car)
  Mux2/1 -> J/1
  Integrator4/1 -> MATLAB Function5/1(x)
  Memory3/1 -> MATLAB Function5/8(aero_coeffs)
  Constant5/1 -> Mux2/2, Mux2/1
  Memory2/1 -> MATLAB Function5/7(F_damp_in)
  MATLAB Function5/7(corner_rh) -> Aeromaps/1(Ride_height)
  MATLAB Function5/5(susp_vel_ground) -> Damper/1(susp_vel_ground)
  Memory5/1 -> MATLAB Function5/2(kin)
  MATLAB Function5/6(IR) -> Damper/2(IR)
  MATLAB Function4/1(Jr_tot) -> MATLAB Function5/6(Jr_tot), Mux2/4, Mux2/3
  <steer>/1 -> kinematics/1(Steer_Angle)
  MATLAB Function5/8(tyre_deflection) -> Bus Creator/3  "tyre_deflection"
  MATLAB Function5/2(Fz) -> Bus Creator1/1  "Fz"
  MATLAB Function5/3(Drag) -> Bus Creator1/2  "Drag"
  Bus Creator1/1 -> [Forces]  "forces"
  Bus Creator/1 -> Bus Creator2/2  "kinematics"
  [Forces] -> Bus Creator2/1  "forces"
  Bus Creator2/1 -> forces & kinematics/1  "forces & kinematics"
  kinematics/1(kin_dyn) -> [kin]
  kinematics/2(anti%) -> [anti]
  [kin] -> Memory5/1
  Damper/1(F_damper) -> [F_damper]
  [F_damper] -> Memory2/1
  Aeromaps/1(aero_coeff) -> [aero]
  [aero] -> Memory3/1
  Veh_States/1 -> Bus Selector/1
  kinematics/3(camber) -> Bus Creator/1  "camber"
  kinematics/4(toe) -> Bus Creator/2  "toe"
  Constant/1 -> Mux/4, Mux/3, Mux/2, Mux/1
  Mux/1 -> kinematics/2(Wheel_Travel)
  MATLAB Function5/9(damping) -> Terminator/1
  Bus Selector/3 -> MATLAB Function5/5(u)  "<u>"
  Bus Selector/2 -> MATLAB Function5/4(ay_prev)  "<ay_prev>"
  Bus Selector/1 -> MATLAB Function5/3(ax_prev)  "<ax_prev>"

== system Vehicle_definitivo_validazione_2/Con relaxation/Vehicle/Powertrain ==
  tps_ICE : Inport
  omega_wheels : Inport  Port=2
  vehicle : Inport  Port=3
  tps_EM : Inport  Port=4
  bps : Inport  Port=5
  Electric Motor : Subsystem
  Mux : Mux
  pwt con clutch : Subsystem  Commented=on
  pwt senza clutch : Subsystem
  gear : Outport
  torque : Outport  Port=2
  wires:
  tps_ICE/1 -> pwt con clutch/1(tps_ICE), pwt senza clutch/1(tps_ICE)  "tps"
  omega_wheels/1 -> pwt senza clutch/4(omega_wheels), pwt con clutch/2(omega_wheels), Electric Motor/2(omega wheels)
  tps_EM/1 -> Electric Motor/1(tps_EM)
  pwt senza clutch/3(gear) -> gear/1
  Electric Motor/1(T_FR) -> Mux/1  "T_FR"
  Electric Motor/2(T_FL) -> Mux/2  "T_FL"
  pwt senza clutch/1(T_RR) -> Mux/3  "T_RR"
  pwt senza clutch/2(T_RL) -> Mux/4  "T_RL"
  Mux/1 -> torque/1  "torque"
  vehicle/1 -> pwt senza clutch/2(vehicle_states), pwt con clutch/3(vehicle_states)
  bps/1 -> pwt con clutch/4(bps), pwt senza clutch/3(bps)

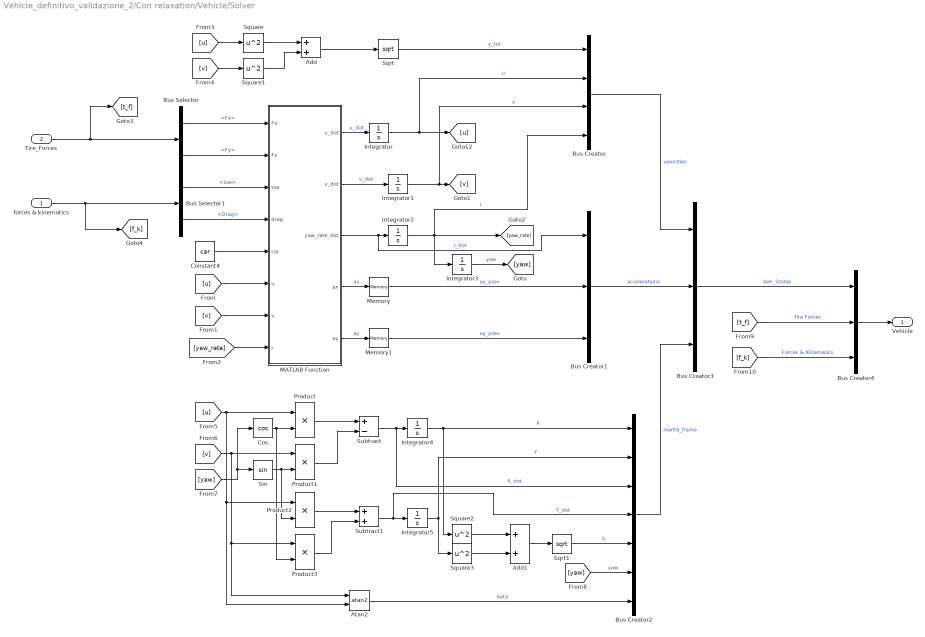
== system Vehicle_definitivo_validazione_2/Con relaxation/Vehicle/Solver ==
  forces & kinematics : Inport
  Tire_Forces : Inport  Port=2
  Add : Sum
  Add1 : Sum
  Atan2 : Trigonometry  Operator=atan2
  Bus Creator : BusCreator  Inputs=4
  Bus Creator1 : BusCreator  Inputs=3
  Bus Creator2 : BusCreator  Inputs=7
  Bus Creator3 : BusCreator  Inputs=3
  Bus Creator4 : BusCreator  Inputs=3
  Bus Selector : BusSelector  OutputSignals=Fx,Fy
  Bus Selector1 : BusSelector  OutputSignals=kinematics.toe,forces.Drag
  Constant4 : Constant  Value=car  OutDataTypeStr=Bus: slBus1
  Cos : Trigonometry  Operator=cos
  Integrator : Integrator  InitialCondition=car.V0
  Integrator{1..5} (5 alike) : Integrator
  MATLAB Function : MATLAB Function  TreatAsAtomicUnit=on
  Memory : Memory
  Memory1 : Memory
  Product{,1..3} (4 alike) : Product
  Sin : Trigonometry
  Sqrt : Sqrt
  Sqrt1 : Sqrt
  Square{,1..3} (4 alike) : Math  Operator=square
  Subtract : Sum  Inputs=+-
  Subtract1 : Sum
  Vehicle : Outport
  wires:
  Subtract/1 -> Bus Creator2/3, Integrator4/1  "X_dot"
  Integrator3/1 -> [yaw]  "yaw"
  [v] -> Atan2/1, Product3/1, Product1/1
  Cos/1 -> Product/2, Product3/2
  MATLAB Function/2(v_dot) -> Integrator1/1  "v_dot"
  Product3/1 -> Subtract1/2
  Integrator5/1 -> Square3/1, Bus Creator2/2  "Y"
  [yaw] -> Cos/1, Sin/1
  Product2/1 -> Subtract1/1
  Integrator4/1 -> Bus Creator2/1, Square2/1  "X"
  MATLAB Function/4(ax) -> Memory/1  "ax"
  [u] -> Product2/1, Atan2/2, Product/1
  [yaw_rate] -> MATLAB Function/8(r)
  Product/1 -> Subtract/1
  Sin/1 -> Product1/2, Product2/2
  Product1/1 -> Subtract/2
  [u] -> MATLAB Function/6(u)
  [v] -> MATLAB Function/7(v)
  MATLAB Function/1(u_dot) -> Integrator/1  "u_dot"
  Subtract1/1 -> Bus Creator2/4, Integrator5/1  "Y_dot"
  MATLAB Function/3(yaw_rate_dot) -> Bus Creator1/1, Integrator2/1  "r_dot"
  Integrator/1 -> [u], Bus Creator/2  "u"
  Memory/1 -> Bus Creator1/2  "ax_prev"
  Memory1/1 -> Bus Creator1/3  "ay_prev"
  Square/1 -> Add/1
  Square1/1 -> Add/2
  Add/1 -> Sqrt/1
  Bus Creator/1 -> Bus Creator3/1  "velocities"
  Bus Creator1/1 -> Bus Creator3/2  "accelerations"
  Bus Creator2/1 -> Bus Creator3/3  "inertia_frame"
  Bus Creator3/1 -> Bus Creator4/1  "Veh_States"
  Constant4/1 -> MATLAB Function/5(car)
  Tire_Forces/1 -> [t_f], Bus Selector/1
  forces & kinematics/1 -> [f_k], Bus Selector1/1
  Bus Selector1/1 -> MATLAB Function/3(toe)  "<toe>"
  Bus Selector1/2 -> MATLAB Function/4(drag)  "<Drag>"
  MATLAB Function/5(ay) -> Memory1/1  "ay"
  Integrator1/1 -> Bus Creator/3, [v]  "v"
  [v] -> Square1/1
  Integrator2/1 -> Bus Creator/4, Integrator3/1, [yaw_rate]  "r"
  Sqrt/1 -> Bus Creator/1  "v_tot"
  [u] -> Square/1
  Square2/1 -> Add1/1
  Square3/1 -> Add1/2
  Add1/1 -> Sqrt1/1
  Sqrt1/1 -> Bus Creator2/5  "S"
  [yaw] -> Bus Creator2/6  "yaw"
  Atan2/1 -> Bus Creator2/7  "beta"
  Bus Selector/2 -> MATLAB Function/2(Fy)  "<Fy>"
  Bus Selector/1 -> MATLAB Function/1(Fx)  "<Fx>"
  [t_f] -> Bus Creator4/2  "Tire Forces"
  [f_k] -> Bus Creator4/3  "Forces & Kinematics"
  Bus Creator4/1 -> Vehicle/1

== system Vehicle_definitivo_validazione_2/Con relaxation/Vehicle/Tyres ==
  forces & kinematics : Inport
  T_motor : Inport  Port=2
  T_brake : Inport  Port=3
  J : Inport  Port=4
  Vehicle : Inport  Port=5
  Bus Creator : BusCreator  Inputs=2
  Bus Selector : BusSelector  OutputSignals=Veh_States.velocities.u,Veh_States.velocities.v,Veh_States.velocities.r
  Bus Selector1 : BusSelector  OutputSignals=kinematics.toe,kinematics.camber,kinematics.tyre_deflection,forces.Fz
  Constant9 : Constant  Value=car  OutDataTypeStr=Bus: slBus1
  Integrator : Integrator
  Integrator1 : Integrator
  Integrator2 : Integrator  InitialCondition=car.V0/car.R
  MATLAB Function : MATLAB Function  TreatAsAtomicUnit=on
  Terminator : Terminator
  Terminator1 : Terminator
  tyres ellisse Adams1 : MATLAB Function  TreatAsAtomicUnit=on
  omega_wheels : Outport
  Tire_Forces : Outport  Port=2
  wires:
  T_motor/1 -> MATLAB Function/3(T_motor)
  Constant9/1 -> tyres ellisse Adams1/1(car)
  J/1 -> MATLAB Function/4(J)
  T_brake/1 -> tyres ellisse Adams1/9(T_brake)
  Bus Creator/1 -> Tire_Forces/1  "Tire_Forces"
  Vehicle/1 -> Bus Selector/1
  forces & kinematics/1 -> Bus Selector1/1
  Bus Selector1/1 -> tyres ellisse Adams1/5(toe)  "<toe>"
  Bus Selector1/2 -> tyres ellisse Adams1/6(camber)  "<camber>"
  Bus Selector1/3 -> tyres ellisse Adams1/7(tyre_deflection)  "<tyre_deflection>"
  Bus Selector1/4 -> tyres ellisse Adams1/8("Fz ")  "<Fz>"
  tyres ellisse Adams1/4(SA) -> Terminator/1  "SA"
  tyres ellisse Adams1/5(SR) -> Terminator1/1  "SR"
  tyres ellisse Adams1/1(Fx_dot) -> Integrator/1  "Fx_dot"
  tyres ellisse Adams1/2(Fy_dot) -> Integrator1/1  "Fy_dot"
  Integrator/1 -> Bus Creator/1, MATLAB Function/1(Fx), tyres ellisse Adams1/11(Fx_dyn)  "Fx"
  Integrator1/1 -> tyres ellisse Adams1/12(Fy_dyn), Bus Creator/2  "Fy"
  tyres ellisse Adams1/6(T_roll) -> MATLAB Function/5(T_roll)  "T_roll"
  tyres ellisse Adams1/7(T_brake_eff) -> MATLAB Function/6(T_brake_eff)  "T_brake_eff"
  tyres ellisse Adams1/8(Rl) -> MATLAB Function/7(Rl)
  MATLAB Function/1(omega_dot) -> Integrator2/1
  Integrator2/1 -> omega_wheels/1, tyres ellisse Adams1/10(omega)
  tyres ellisse Adams1/3(Fz) -> MATLAB Function/2(Fz)
  Bus Selector/3 -> tyres ellisse Adams1/4(r)  "<r>"
  Bus Selector/2 -> tyres ellisse Adams1/3(v)  "<v>"
  Bus Selector/1 -> tyres ellisse Adams1/2(u)  "<u>"

== system Vehicle_definitivo_validazione_2/Driver in the Loop/Vehicle/Brakes ==
  BP_tot : Inport
  Constant : Constant  Value=car.bp_max
  Front Caliper : Subsystem
  Gain : Gain  Gain=car.brakebias
  Gain1 : Gain  Gain=1-car.brakebias
  Mux : Mux
  Product2 : Product
  Proportional Valve : Subsystem
  Rear Caliper : Subsystem
  Brake_torque : Outport
  wires:
  Gain/1 -> Front Caliper/1(P_Front)
  Proportional Valve/1(p_rear_mod) -> Rear Caliper/1(P_rear)
  Gain1/1 -> Proportional Valve/1(P_rear)
  Product2/1 -> Gain1/1, Gain/1
  Rear Caliper/1(T_brake_RR) -> Mux/3  "T_brake_RR"
  Rear Caliper/2(T_brake_RL) -> Mux/4  "T_brake_RL"
  Mux/1 -> Brake_torque/1  "Brake_Torque"
  BP_tot/1 -> Product2/1
  Constant/1 -> Product2/2
  Front Caliper/2(T_brake_FL) -> Mux/2  "T_brake_FL"
  Front Caliper/1(T_brake_FR) -> Mux/1  "T_brake_FR"

== system Vehicle_definitivo_validazione_2/Driver in the Loop/Vehicle/Chassis ==
  Veh_States : Inport
  <steer> : Inport  Port=2
  gear : Inport  Port=3
  Aeromaps : Subsystem
  Bus Creator : BusCreator  Inputs=3
  Bus Creator1 : BusCreator  Inputs=2
  Bus Creator2 : BusCreator  Inputs=2
  Bus Selector : BusSelector  OutputSignals=Veh_States.accelerations.ax_prev,Veh_States.accelerations.ay_prev,Veh_States.velocities.u
  Constant : Constant  Value=0
  Constant12 : Constant  Value=car  OutDataTypeStr=Bus: slBus1
  Constant5 : Constant  Value=car.J_f
  Damper : Subsystem
  Integrator4 : Integrator  InitialCondition=zeros(14,1)
  MATLAB Function4 : MATLAB Function  TreatAsAtomicUnit=on
  MATLAB Function5 : MATLAB Function  TreatAsAtomicUnit=on
  Memory2 : Memory  InheritSampleTime=on
  Memory3 : Memory  InitialCondition=[car.Cz, car.Cx, car.x_cp]  InheritSampleTime=on
  Memory5 : Memory  InitialCondition=[car.IR_spring_front, car.IR_spring_front, car.IR_spring_rear, car.IR_spring_rear, car.tf, car.tr, car.lf, car.lr, car.h_cog, 0.03, 0.04]  InheritSampleTime=on
  Mux : Mux
  Mux2 : Mux
  Terminator : Terminator
  kinematics : Subsystem
  forces & kinematics : Outport
  J : Outport  Port=2
  wires:
  MATLAB Function5/1(dx) -> Integrator4/1
  gear/1 -> MATLAB Function4/1(gear)
  Constant12/1 -> MATLAB Function4/2(car), MATLAB Function5/9(car)
  Mux2/1 -> J/1
  Integrator4/1 -> MATLAB Function5/1(x)
  Memory3/1 -> MATLAB Function5/8(aero_coeffs)
  Constant5/1 -> Mux2/2, Mux2/1
  Memory2/1 -> MATLAB Function5/7(F_damp_in)
  MATLAB Function5/7(corner_rh) -> Aeromaps/1(Ride_height)
  MATLAB Function5/5(susp_vel_ground) -> Damper/1(susp_vel_ground)
  Memory5/1 -> MATLAB Function5/2(kin)
  MATLAB Function5/6(IR) -> Damper/2(IR)
  MATLAB Function4/1(Jr_tot) -> MATLAB Function5/6(Jr_tot), Mux2/4, Mux2/3
  <steer>/1 -> kinematics/1(Steer_Angle)
  MATLAB Function5/8(tyre_deflection) -> Bus Creator/3  "tyre_deflection"
  MATLAB Function5/2(Fz) -> Bus Creator1/1  "Fz"
  MATLAB Function5/3(Drag) -> Bus Creator1/2  "Drag"
  Bus Creator1/1 -> [Forces]  "forces"
  Bus Creator/1 -> Bus Creator2/2  "kinematics"
  [Forces] -> Bus Creator2/1  "forces"
  Bus Creator2/1 -> forces & kinematics/1  "forces & kinematics"
  kinematics/1(kin_dyn) -> [kin]
  kinematics/2(anti%) -> [anti]
  [kin] -> Memory5/1
  Damper/1(F_damper) -> [F_damper]
  [F_damper] -> Memory2/1
  Aeromaps/1(aero_coeff) -> [aero]
  [aero] -> Memory3/1
  Veh_States/1 -> Bus Selector/1
  kinematics/3(camber) -> Bus Creator/1  "camber"
  kinematics/4(toe) -> Bus Creator/2  "toe"
  Constant/1 -> Mux/4, Mux/3, Mux/2, Mux/1
  Mux/1 -> kinematics/2(Wheel_Travel)
  MATLAB Function5/9(damping) -> Terminator/1
  Bus Selector/3 -> MATLAB Function5/5(u)  "<u>"
  Bus Selector/2 -> MATLAB Function5/4(ay_prev)  "<ay_prev>"
  Bus Selector/1 -> MATLAB Function5/3(ax_prev)  "<ax_prev>"

== system Vehicle_definitivo_validazione_2/Driver in the Loop/Vehicle/Powertrain ==
  tps_ICE : Inport
  omega_wheels : Inport  Port=2
  vehicle : Inport  Port=3
  tps_EM : Inport  Port=4
  bps : Inport  Port=5
  Electric Motor : Subsystem
  Mux : Mux
  pwt con clutch : Subsystem  Commented=on
  pwt senza clutch : Subsystem
  gear : Outport
  torque : Outport  Port=2
  wires:
  tps_ICE/1 -> pwt con clutch/1(tps_ICE), pwt senza clutch/1(tps_ICE)  "tps"
  omega_wheels/1 -> pwt senza clutch/4(omega_wheels), pwt con clutch/2(omega_wheels), Electric Motor/2(omega wheels)
  tps_EM/1 -> Electric Motor/1(tps_EM)
  pwt senza clutch/3(gear) -> gear/1
  Electric Motor/1(T_FR) -> Mux/1  "T_FR"
  Electric Motor/2(T_FL) -> Mux/2  "T_FL"
  pwt senza clutch/1(T_RR) -> Mux/3  "T_RR"
  pwt senza clutch/2(T_RL) -> Mux/4  "T_RL"
  Mux/1 -> torque/1  "torque"
  vehicle/1 -> pwt senza clutch/2(vehicle_states), pwt con clutch/3(vehicle_states)
  bps/1 -> pwt con clutch/4(bps), pwt senza clutch/3(bps)

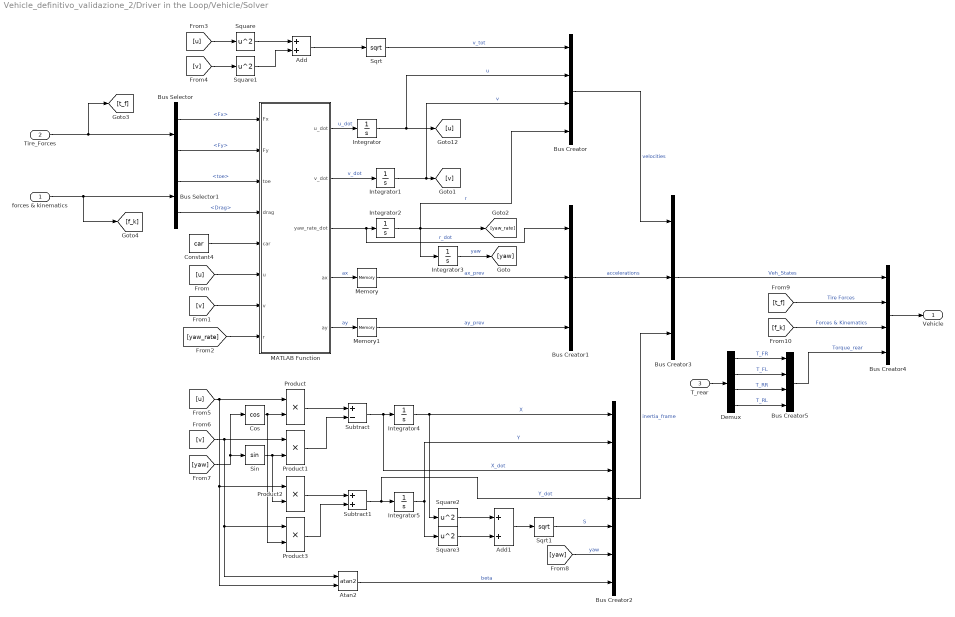
== system Vehicle_definitivo_validazione_2/Driver in the Loop/Vehicle/Solver ==
  forces & kinematics : Inport
  Tire_Forces : Inport  Port=2
  T_rear : Inport  Port=3
  Add : Sum
  Add1 : Sum
  Atan2 : Trigonometry  Operator=atan2
  Bus Creator : BusCreator  Inputs=4
  Bus Creator1 : BusCreator  Inputs=3
  Bus Creator2 : BusCreator  Inputs=7
  Bus Creator3 : BusCreator  Inputs=3
  Bus Creator4 : BusCreator  Inputs=4
  Bus Creator5 : BusCreator  Inputs=4
  Bus Selector : BusSelector  OutputSignals=Fx,Fy
  Bus Selector1 : BusSelector  OutputSignals=kinematics.toe,forces.Drag
  Constant4 : Constant  Value=car  OutDataTypeStr=Bus: slBus1
  Cos : Trigonometry  Operator=cos
  Demux : Demux
  Integrator : Integrator  InitialCondition=car.V0
  Integrator{1..5} (5 alike) : Integrator
  MATLAB Function : MATLAB Function  TreatAsAtomicUnit=on
  Memory : Memory
  Memory1 : Memory
  Product{,1..3} (4 alike) : Product
  Sin : Trigonometry
  Sqrt : Sqrt
  Sqrt1 : Sqrt
  Square{,1..3} (4 alike) : Math  Operator=square
  Subtract : Sum  Inputs=+-
  Subtract1 : Sum
  Vehicle : Outport
  wires:
  Subtract/1 -> Bus Creator2/3, Integrator4/1  "X_dot"
  Integrator3/1 -> [yaw]  "yaw"
  [v] -> Atan2/1, Product3/1, Product1/1
  Cos/1 -> Product/2, Product3/2
  MATLAB Function/2(v_dot) -> Integrator1/1  "v_dot"
  Product3/1 -> Subtract1/2
  Integrator5/1 -> Square3/1, Bus Creator2/2  "Y"
  [yaw] -> Cos/1, Sin/1
  Product2/1 -> Subtract1/1
  Integrator4/1 -> Bus Creator2/1, Square2/1  "X"
  MATLAB Function/4(ax) -> Memory/1  "ax"
  [u] -> Product2/1, Atan2/2, Product/1
  [yaw_rate] -> MATLAB Function/8(r)
  Product/1 -> Subtract/1
  Sin/1 -> Product1/2, Product2/2
  Product1/1 -> Subtract/2
  [u] -> MATLAB Function/6(u)
  [v] -> MATLAB Function/7(v)
  MATLAB Function/1(u_dot) -> Integrator/1  "u_dot"
  Subtract1/1 -> Bus Creator2/4, Integrator5/1  "Y_dot"
  MATLAB Function/3(yaw_rate_dot) -> Bus Creator1/1, Integrator2/1  "r_dot"
  Integrator/1 -> [u], Bus Creator/2  "u"
  Memory/1 -> Bus Creator1/2  "ax_prev"
  Memory1/1 -> Bus Creator1/3  "ay_prev"
  Square/1 -> Add/1
  Square1/1 -> Add/2
  Add/1 -> Sqrt/1
  Bus Creator/1 -> Bus Creator3/1  "velocities"
  Bus Creator1/1 -> Bus Creator3/2  "accelerations"
  Bus Creator2/1 -> Bus Creator3/3  "inertia_frame"
  Bus Creator3/1 -> Bus Creator4/1  "Veh_States"
  Constant4/1 -> MATLAB Function/5(car)
  Tire_Forces/1 -> [t_f], Bus Selector/1
  forces & kinematics/1 -> [f_k], Bus Selector1/1
  Bus Selector1/1 -> MATLAB Function/3(toe)  "<toe>"
  Bus Selector1/2 -> MATLAB Function/4(drag)  "<Drag>"
  MATLAB Function/5(ay) -> Memory1/1  "ay"
  Integrator1/1 -> Bus Creator/3, [v]  "v"
  [v] -> Square1/1
  Integrator2/1 -> Bus Creator/4, Integrator3/1, [yaw_rate]  "r"
  Sqrt/1 -> Bus Creator/1  "v_tot"
  [u] -> Square/1
  Square2/1 -> Add1/1
  Square3/1 -> Add1/2
  Add1/1 -> Sqrt1/1
  Sqrt1/1 -> Bus Creator2/5  "S"
  [yaw] -> Bus Creator2/6  "yaw"
  Atan2/1 -> Bus Creator2/7  "beta"
  Bus Selector/2 -> MATLAB Function/2(Fy)  "<Fy>"
  Bus Selector/1 -> MATLAB Function/1(Fx)  "<Fx>"
  [t_f] -> Bus Creator4/2  "Tire Forces"
  [f_k] -> Bus Creator4/3  "Forces & Kinematics"
  Bus Creator4/1 -> Vehicle/1
  T_rear/1 -> Demux/1
  Bus Creator5/1 -> Bus Creator4/4  "Torque_rear"
  Demux/3 -> Bus Creator5/3  "T_RR"
  Demux/4 -> Bus Creator5/4  "T_RL"
  Demux/1 -> Bus Creator5/1  "T_FR"
  Demux/2 -> Bus Creator5/2  "T_FL"
